simulink model "Sim_CVBT"  (R2022a)
settings: Solver=ode45  StartTime=0.0  StopTime=600  FixedStep=0.01  RelTol=1e-3  EnableMultiTasking=on
InitFcn:
  | initialize;
  | %graphics_init;
values from neighbouring files (symbols this model uses):
  a = 0.08    [initialize.m]
  b = 0.002*0    (= 0)    [initialize.m]
  Kdv = 0    [initialize.m]
  Kiv = 0    [initialize.m]
  Kpsi = 2    [initialize.m]
  Kpv = 0.2    [initialize.m]
  numVeh = 6    [initialize.m]
  P0 = zeros(40,1)    [initialize.m]
  P0tg = [-400 -400 0]    [initialize.m]
  psi0 = zeros(20,1)    [initialize.m]
  rho_d = [100 150 100 150 100 150 100 150 100 150]    [initialize.m]
  Vg = zeros(10,1)    [initialize.m]
  Vmax = 60    [initialize.m]
  Vmin = 10    [initialize.m]
  z0 = zeros(20,1)    [initialize.m]
libraries: slpidlib x6, simulink x2
(part 2 of 2)

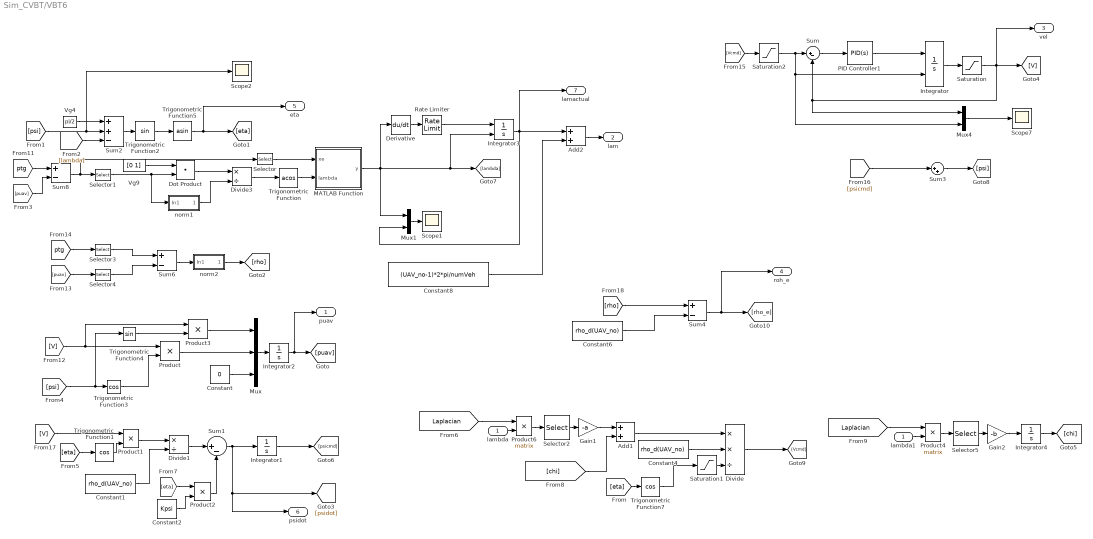
== system Sim_CVBT/VBT6 ==
  lambda : Inport
  Add1 : Sum
  Add2 : Sum
  Constant : Constant  Value=0
  Constant1 : Constant  Value=rho_d(UAV_no)
  Constant2 : Constant  Value=Kpsi
  Constant4 : Constant  Value=rho_d(UAV_no)
  Constant6 : Constant  Value=rho_d(UAV_no)
  Constant8 : Constant  Value=(UAV_no-1)*2*pi/numVeh
  Derivative : Derivative
  Divide : Product  Inputs=**/
  Divide1 : Product  Inputs=*/
  Divide3 : Product  Inputs=*/
  Dot Product : DotProduct  OutDataTypeStr=Inherit: Inherit via internal rule
  Gain1 : Gain  Gain=-a
  Gain2 : Gain  Gain=-b
  Integrator : Integrator  InitialConditionSource=external
  Integrator1 : Integrator  InitialCondition=psi0(UAV_no)*pi/180
  Integrator2 : Integrator  InitialCondition=[P0(2*UAV_no-1) P0(2*UAV_no) z0(UAV_no)]
  Integrator3 : Integrator  InitialConditionSource=external
  Integrator4 : Integrator  InitialCondition=Vg(UAV_no)/rho_d(UAV_no)
  MATLAB Function : MATLAB Function  TreatAsAtomicUnit=on
  Mux : Mux  Inputs=3
  Mux1 : Mux  Inputs=2
  Mux4 : Mux  Inputs=2
  PID Controller1 : slpidlib/PID Controller  Controller=PID  Form=Parallel  TimeDomain=Continuous-time  UseExternalTs=off  SampleTime=1  IntegratorMethod=Forward Euler  FilterMethod=Forward Euler  ControllerParametersSource=internal  P=Kpv  I=Kiv  UseKiTs=off  D=Kdv  N=100  UseFilter=on  TunerSelectOption=Transfer Function Based (PID Tuner App)  InitialConditionSource=internal  InitialConditionForIntegrator=0  InitialConditionForFilter=0  DifferentiatorICPrevScaledInput=0  ExternalReset=none  TrackingMode=off  Kt=1  LimitOutput=off  SatLimitsSource=internal  UpperSaturationLimit=inf  LowerSaturationLimit=-inf  LinearizeAsGain=on  AntiWindupMode=none  Kb=1  POutMin=[]  POutMax=[]  IOutMin=[]  IOutMax=[]  DOutMin=[]  DOutMax=[]  NOutMin=[]  NOutMax=[]  SumOutMin=[]  SumOutMax=[]  SaturationOutMin=[]  SaturationOutMax=[]  PParamMin=[]  PParamMax=[]  IParamMin=[]  IParamMax=[]  DParamMin=[]  DParamMax=[]  NParamMin=[]  NParamMax=[]  KbParamMin=[]  KbParamMax=[]  KtParamMin=[]  KtParamMax=[]  KbOutMin=[]  KbOutMax=[]  KtOutMin=[]  KtOutMax=[]  IntegratorOutMin=[]  IntegratorOutMax=[]  FilterOutMin=[]  FilterOutMax=[]  SumI1OutMin=[]  SumI1OutMax=[]  SumI2OutMin=[]  SumI2OutMax=[]  SumI3OutMin=[]  SumI3OutMax=[]  SumI4OutMin=[]  SumI4OutMax=[]  SumDOutMin=[]  SumDOutMax=[]  DifferentiatorOutMin=[]  DifferentiatorOutMax=[]  FilterDiffOutCoefMin=[]  FilterDiffOutCoefMax=[]  ReciprocalOutMin=[]  ReciprocalOutMax=[]  SumDenOutMin=[]  SumDenOutMax=[]  SumNumOutMin=[]  SumNumOutMax=[]  DivideOutMin=[]  DivideOutMax=[]  UdiffTsProdOutMin=[]  UdiffTsProdOutMax=[]  NTsProdOutMin=[]  NTsProdOutMax=[]  UintegralTsProdOutMin=[]  UintegralTsProdOutMax=[]  UngainTsProdOutMin=[]  UngainTsProdOutMax=[]  IntegratorContinuousStateAttributes=''  IntegratorStateMustResolveToSignalObject=off  IntegratorRTWStateStorageClass=Auto  FilterContinuousStateAttributes=''  FilterStateMustResolveToSignalObject=off  FilterRTWStateStorageClass=Auto  ParallelPVariant=InternalParameters  IdealPVariant=Disabled  IVariant=InternalParameters  DVariant=InternalParameters  IntegratorVariant=Continuous  SatVariant=Disabled  AWVariant=Passthrough  PCopyVariant=Disabled  TRVariant=Disabled  FdbkBlocksVariant=Forward  IdealPFdbkVariant=Disabled  SatFdbkVariant=Disabled  DerivativeFilterVariant=ContFilter  NVariant=InternalParameters  NCopyVariant=Disabled  FilterICVariant=InternalICsFilter  IntegratorICVariant=InternalICs  ExternalResetVariant=Disabled  TRSumVariant=Passthrough  SumFdbkVariant=Disabled  SumVariant=Sum_PID  TsampFilterVariant=InternalTs  TsampNgainVariant=Passthrough  TsampIntegralVariant=Passthrough  ExternalSaturationOutDataTypeStr=Inherit: Same as second input  aMode=0
  Product{,1..3} (4 alike) : Product  RndMeth=Zero
  Product4 : Product  Multiplication=Matrix(*)  RndMeth=Zero
  Product6 : Product  Multiplication=Matrix(*)  RndMeth=Zero
  Rate Limiter : RateLimiter  RisingSlewLimit=100  FallingSlewLimit=-0.1  SampleTimeMode=inherited
  Saturation : Saturate  UpperLimit=Vmax  LowerLimit=Vmin
  Saturation1 : Saturate  UpperLimit=1  LowerLimit=0.8
  Saturation2 : Saturate  UpperLimit=Vmax  LowerLimit=Vmin
  Scope1 : Scope
  Scope2 : Scope
  Scope7 : Scope
  Selector : Selector  InputPortWidth=3  IndexOptions=Index vector (dialog)  Indices=1  OutputSizes=1
  Selector1 : Selector  InputPortWidth=3  IndexOptions=Index vector (dialog)  Indices=[1 2]  OutputSizes=1
  Selector2 : Selector  InputPortWidth=6  IndexOptions=Index vector (dialog)  Indices=[UAV_no]  OutputSizes=1
  Selector3 : Selector  InputPortWidth=3  IndexOptions=Index vector (dialog)  Indices=[1 2]  OutputSizes=1
  Selector4 : Selector  InputPortWidth=3  IndexOptions=Index vector (dialog)  Indices=[1 2]  OutputSizes=1
  Selector5 : Selector  InputPortWidth=6  IndexOptions=Index vector (dialog)  Indices=[UAV_no]  OutputSizes=1
  Sum : Sum  Inputs=|+-
  Sum1 : Sum  Inputs=|+-
  Sum2 : Sum  Inputs=++-
  Sum3 : Sum  Inputs=|++
  Sum4 : Sum  Inputs=+-
  Sum6 : Sum  Inputs=+-
  Sum8 : Sum  Inputs=+-
  Trigonometric Function : Trigonometry  Operator=acos
  Trigonometric Function1 : Trigonometry  Operator=cos
  Trigonometric Function2 : Trigonometry
  Trigonometric Function3 : Trigonometry  Operator=cos
  Trigonometric Function4 : Trigonometry
  Trigonometric Function5 : Trigonometry  Operator=asin
  Trigonometric Function7 : Trigonometry  Operator=cos
  Vg4 : Constant  Value=pi/2
  Vg9 : Constant  Value=[0 1]
  lambda1 : InportShadow
  norm1 : Subsystem
  norm2 : Subsystem
  puav : Outport
  lam : Outport  Port=2
  vel : Outport  Port=3
  roh_e : Outport  Port=4
  eta : Outport  Port=5
  psidot : Outport  Port=6
  lamactual : Outport  Port=7
  wires:
  Mux4/1 -> Scope7/1
  PID Controller1/1 -> Integrator/1
  Integrator/1 -> Saturation/1
  Saturation/1 -> Mux4/1, Sum/2, [V], vel/1
  Saturation1/1 -> Divide/3
  Sum4/1 -> [rho_e], roh_e/1
  Constant6/1 -> Sum4/2
  [rho] -> Sum4/1
  Sum3/1 -> [psi]
  [psicmd] -> Sum3/1
  [Vcmd] -> Saturation2/1
  Sum/1 -> PID Controller1/1
  Constant8/1 -> Add2/2
  Add2/1 -> lam/1
  Integrator3/1 -> lamactual/1, Mux1/2, Add2/1
  Derivative/1 -> Rate Limiter/1
  MATLAB Function/1(y) -> [lambda], Integrator3/2, Mux1/1, Derivative/1
  Divide3/1 -> Trigonometric Function/1
  Trigonometric Function/1 -> MATLAB Function/2(lambda)
  Selector4/1 -> Sum6/2
  Selector3/1 -> Sum6/1
  Selector2/1 -> Gain1/1
  Divide/1 -> [Vcmd]
  lambda/1 -> Product6/2
  [Laplacian] -> Product6/1
  Product6/1 -> Selector2/1
  Constant4/1 -> Divide/2
  Trigonometric Function7/1 -> Saturation1/1
  Gain1/1 -> Add1/1
  Add1/1 -> Divide/1
  [eta] -> Trigonometric Function7/1
  Mux1/1 -> Scope1/1
  [V] -> Product1/1
  norm2/1(Out1) -> [rho]
  Selector1/1 -> norm1/1(In1), Dot Product/2
  Integrator2/1 -> [puav], puav/1
  Mux/1 -> Integrator2/1
  Constant/1 -> Mux/3
  Product/1 -> Mux/2
  Product3/1 -> Mux/1
  Trigonometric Function4/1 -> Product3/2
  Trigonometric Function3/1 -> Product/2
  [psi] -> Trigonometric Function4/1, Trigonometric Function3/1
  [V] -> Product3/1, Product/1
  Trigonometric Function5/1 -> [eta], eta/1
  Trigonometric Function2/1 -> Trigonometric Function5/1
  Vg9/1 -> Dot Product/1
  Selector/1 -> MATLAB Function/1(xe)
  Integrator1/1 -> [psicmd]
  [puav] -> Sum8/2
  [ptg] -> Sum8/1
  norm1/1(Out1) -> Divide3/2
  Dot Product/1 -> Divide3/1
  [lambda] -> Sum2/3
  [psi] -> Sum2/2, Scope2/1
  Sum8/1 -> Selector1/1, Selector/1
  Vg4/1 -> Sum2/1
  Sum2/1 -> Trigonometric Function2/1
  [ptg] -> Selector3/1
  [puav] -> Selector4/1
  Sum6/1 -> norm2/1(In1)
  Sum1/1 -> [psidot], psidot/1, Integrator1/1
  Constant2/1 -> Product2/2
  Product2/1 -> Sum1/2
  [eta] -> Product2/1
  Constant1/1 -> Divide1/2
  Product1/1 -> Divide1/1
  Divide1/1 -> Sum1/1
  [eta] -> Trigonometric Function1/1
  Trigonometric Function1/1 -> Product1/2
  Rate Limiter/1 -> Integrator3/1
  [chi] -> Add1/2
  Selector5/1 -> Gain2/1
  lambda1/1 -> Product4/2
  [Laplacian] -> Product4/1
  Product4/1 -> Selector5/1
  Gain2/1 -> Integrator4/1
  Integrator4/1 -> [chi]
  Saturation2/1 -> Sum/1, Integrator/2, Mux4/2

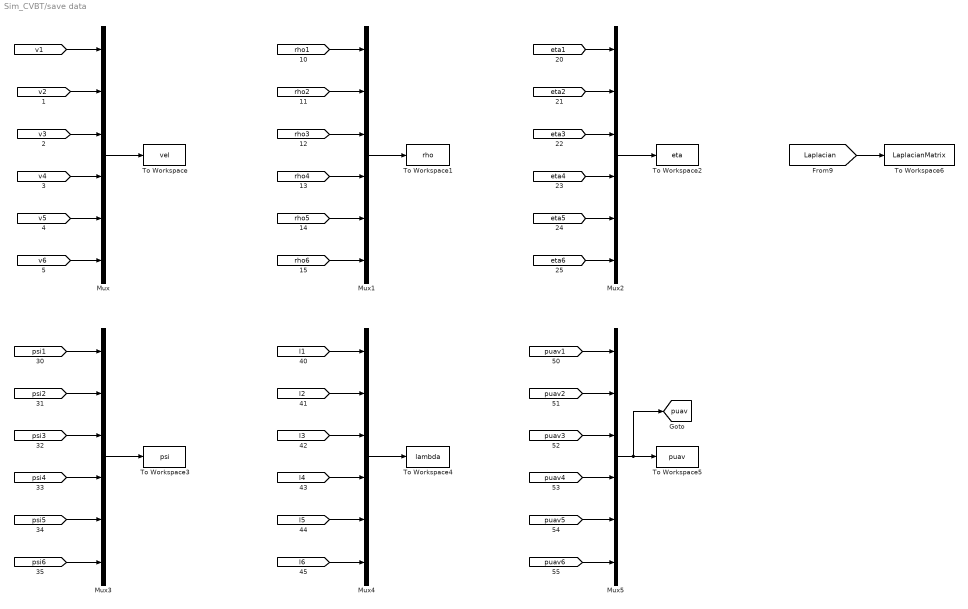
== system Sim_CVBT/save data ==
  Mux{,1..5} (6 alike) : Mux  Inputs=6
  To Workspace : ToWorkspace  VariableName=vel  SaveFormat=Timeseries  SampleTime=-1
  To Workspace1 : ToWorkspace  VariableName=rho  SaveFormat=Timeseries  SampleTime=-1
  To Workspace2 : ToWorkspace  VariableName=eta  SaveFormat=Timeseries  SampleTime=-1
  To Workspace3 : ToWorkspace  VariableName=psi  SaveFormat=Timeseries  SampleTime=-1
  To Workspace4 : ToWorkspace  VariableName=lambda  SaveFormat=Timeseries  SampleTime=-1
  To Workspace5 : ToWorkspace  VariableName=puav  SaveFormat=Timeseries  SampleTime=-1
  To Workspace6 : ToWorkspace  VariableName=LaplacianMatrix  SaveFormat=Timeseries  SampleTime=-1
  tag scope: puav=global
  wires:
  [v1] -> Mux/1
  [v3] -> Mux/3
  [v6] -> Mux/6
  [v5] -> Mux/5
  [v4] -> Mux/4
  [v2] -> Mux/2
  [rho3] -> Mux1/3
  [rho6] -> Mux1/6
  [rho5] -> Mux1/5
  [rho4] -> Mux1/4
  [rho2] -> Mux1/2
  [rho1] -> Mux1/1
  [eta3] -> Mux2/3
  [eta6] -> Mux2/6
  [eta5] -> Mux2/5
  [eta4] -> Mux2/4
  [eta2] -> Mux2/2
  [eta1] -> Mux2/1
  [psi3] -> Mux3/3
  [psi6] -> Mux3/6
  [psi5] -> Mux3/5
  [psi4] -> Mux3/4
  [psi2] -> Mux3/2
  [psi1] -> Mux3/1
  [l3] -> Mux4/3
  [l6] -> Mux4/6
  [l5] -> Mux4/5
  [l4] -> Mux4/4
  [l2] -> Mux4/2
  [l1] -> Mux4/1
  Mux/1 -> To Workspace/1
  Mux1/1 -> To Workspace1/1
  Mux2/1 -> To Workspace2/1
  Mux3/1 -> To Workspace3/1
  Mux4/1 -> To Workspace4/1
  [puav3] -> Mux5/3
  [puav6] -> Mux5/6
  [puav5] -> Mux5/5
  [puav4] -> Mux5/4
  [puav2] -> Mux5/2
  [puav1] -> Mux5/1
  Mux5/1 -> [puav], To Workspace5/1
  [Laplacian] -> To Workspace6/1

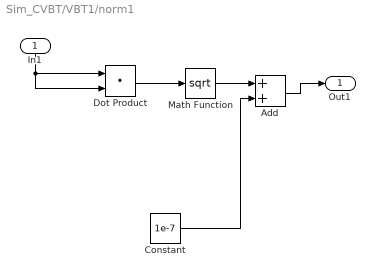
== system Sim_CVBT/VBT1/norm1 ==
  In1 : Inport
  Add : Sum
  Constant : Constant  Value=1e-7
  Dot Product : DotProduct  OutDataTypeStr=Inherit: Inherit via internal rule
  Math Function : Math  Operator=sqrt  SignedPower=on
  Out1 : Outport
  wires:
  Dot Product/1 -> Math Function/1
  In1/1 -> Dot Product/1, Dot Product/2
  Math Function/1 -> Add/1
  Constant/1 -> Add/2
  Add/1 -> Out1/1

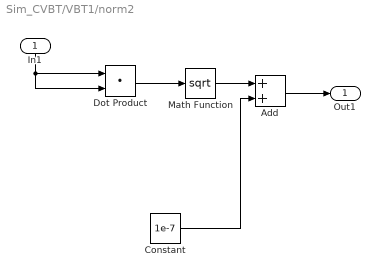
== system Sim_CVBT/VBT1/norm2 ==
  In1 : Inport
  Add : Sum
  Constant : Constant  Value=1e-7
  Dot Product : DotProduct  OutDataTypeStr=Inherit: Inherit via internal rule
  Math Function : Math  Operator=sqrt  SignedPower=on
  Out1 : Outport
  wires:
  Add/1 -> Out1/1
  Constant/1 -> Add/2
  Math Function/1 -> Add/1
  In1/1 -> Dot Product/2, Dot Product/1
  Dot Product/1 -> Math Function/1

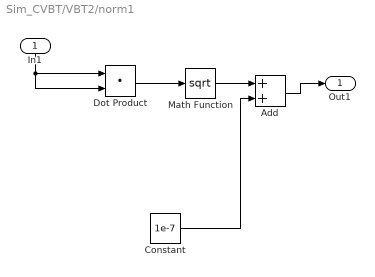
== system Sim_CVBT/VBT2/norm1 ==
  In1 : Inport
  Add : Sum
  Constant : Constant  Value=1e-7
  Dot Product : DotProduct  OutDataTypeStr=Inherit: Inherit via internal rule
  Math Function : Math  Operator=sqrt  SignedPower=on
  Out1 : Outport
  wires:
  Add/1 -> Out1/1
  Constant/1 -> Add/2
  Math Function/1 -> Add/1
  In1/1 -> Dot Product/2, Dot Product/1
  Dot Product/1 -> Math Function/1

== system Sim_CVBT/VBT2/norm2 ==
  In1 : Inport
  Add : Sum
  Constant : Constant  Value=1e-7
  Dot Product : DotProduct  OutDataTypeStr=Inherit: Inherit via internal rule
  Math Function : Math  Operator=sqrt  SignedPower=on
  Out1 : Outport
  wires:
  Dot Product/1 -> Math Function/1
  In1/1 -> Dot Product/1, Dot Product/2
  Math Function/1 -> Add/1
  Constant/1 -> Add/2
  Add/1 -> Out1/1

== system Sim_CVBT/VBT3/norm1 ==
  In1 : Inport
  Add : Sum
  Constant : Constant  Value=1e-7
  Dot Product : DotProduct  OutDataTypeStr=Inherit: Inherit via internal rule
  Math Function : Math  Operator=sqrt  SignedPower=on
  Out1 : Outport
  wires:
  Dot Product/1 -> Math Function/1
  In1/1 -> Dot Product/1, Dot Product/2
  Math Function/1 -> Add/1
  Constant/1 -> Add/2
  Add/1 -> Out1/1

== system Sim_CVBT/VBT3/norm2 ==
  In1 : Inport
  Add : Sum
  Constant : Constant  Value=1e-7
  Dot Product : DotProduct  OutDataTypeStr=Inherit: Inherit via internal rule
  Math Function : Math  Operator=sqrt  SignedPower=on
  Out1 : Outport
  wires:
  Add/1 -> Out1/1
  Constant/1 -> Add/2
  Math Function/1 -> Add/1
  In1/1 -> Dot Product/2, Dot Product/1
  Dot Product/1 -> Math Function/1

== system Sim_CVBT/VBT4/norm1 ==
  In1 : Inport
  Add : Sum
  Constant : Constant  Value=1e-7
  Dot Product : DotProduct  OutDataTypeStr=Inherit: Inherit via internal rule
  Math Function : Math  Operator=sqrt  SignedPower=on
  Out1 : Outport
  wires:
  Add/1 -> Out1/1
  Constant/1 -> Add/2
  Math Function/1 -> Add/1
  In1/1 -> Dot Product/2, Dot Product/1
  Dot Product/1 -> Math Function/1

== system Sim_CVBT/VBT4/norm2 ==
  In1 : Inport
  Add : Sum
  Constant : Constant  Value=1e-7
  Dot Product : DotProduct  OutDataTypeStr=Inherit: Inherit via internal rule
  Math Function : Math  Operator=sqrt  SignedPower=on
  Out1 : Outport
  wires:
  Dot Product/1 -> Math Function/1
  In1/1 -> Dot Product/1, Dot Product/2
  Math Function/1 -> Add/1
  Constant/1 -> Add/2
  Add/1 -> Out1/1

== system Sim_CVBT/VBT5/norm1 ==
  In1 : Inport
  Add : Sum
  Constant : Constant  Value=1e-7
  Dot Product : DotProduct  OutDataTypeStr=Inherit: Inherit via internal rule
  Math Function : Math  Operator=sqrt  SignedPower=on
  Out1 : Outport
  wires:
  Dot Product/1 -> Math Function/1
  In1/1 -> Dot Product/1, Dot Product/2
  Math Function/1 -> Add/1
  Constant/1 -> Add/2
  Add/1 -> Out1/1

== system Sim_CVBT/VBT5/norm2 ==
  In1 : Inport
  Add : Sum
  Constant : Constant  Value=1e-7
  Dot Product : DotProduct  OutDataTypeStr=Inherit: Inherit via internal rule
  Math Function : Math  Operator=sqrt  SignedPower=on
  Out1 : Outport
  wires:
  Add/1 -> Out1/1
  Constant/1 -> Add/2
  Math Function/1 -> Add/1
  In1/1 -> Dot Product/2, Dot Product/1
  Dot Product/1 -> Math Function/1

== system Sim_CVBT/VBT6/norm1 ==
  In1 : Inport
  Add : Sum
  Constant : Constant  Value=1e-7
  Dot Product : DotProduct  OutDataTypeStr=Inherit: Inherit via internal rule
  Math Function : Math  Operator=sqrt  SignedPower=on
  Out1 : Outport
  wires:
  Add/1 -> Out1/1
  Constant/1 -> Add/2
  Math Function/1 -> Add/1
  In1/1 -> Dot Product/2, Dot Product/1
  Dot Product/1 -> Math Function/1

== system Sim_CVBT/VBT6/norm2 ==
  In1 : Inport
  Add : Sum
  Constant : Constant  Value=1e-7
  Dot Product : DotProduct  OutDataTypeStr=Inherit: Inherit via internal rule
  Math Function : Math  Operator=sqrt  SignedPower=on
  Out1 : Outport
  wires:
  Dot Product/1 -> Math Function/1
  In1/1 -> Dot Product/1, Dot Product/2
  Math Function/1 -> Add/1
  Constant/1 -> Add/2
  Add/1 -> Out1/1

== matlab function Sim_CVBT/VBT1/MATLAB Function ==
  data: xe input; y output; lambda input
function y = fcn(xe,lambda)
u=lambda;
if xe > 0 
    u = lambda;
else
    u = 2*pi-lambda;
end
y = u;

== matlab function Sim_CVBT/VBT2/MATLAB Function ==
  data: xe input; y output; lambda input
function y = fcn(xe,lambda)
u=lambda;
if xe > 0 
    u = lambda;
else
    u = 2*pi-lambda;
end
y = u;

== matlab function Sim_CVBT/VBT3/MATLAB Function ==
  data: xe input; y output; lambda input
function y = fcn(xe,lambda)
u=lambda;
if xe > 0 
    u = lambda;
else
    u = 2*pi-lambda;
end
y = u;

== matlab function Sim_CVBT/VBT4/MATLAB Function ==
  data: xe input; y output; lambda input
function y = fcn(xe,lambda)
u=lambda;
if xe > 0 
    u = lambda;
else
    u = 2*pi-lambda;
end
y = u;

== matlab function Sim_CVBT/VBT5/MATLAB Function ==
  data: xe input; y output; lambda input
function y = fcn(xe,lambda)
u=lambda;
if xe > 0 
    u = lambda;
else
    u = 2*pi-lambda;
end
y = u;

== matlab function Sim_CVBT/VBT6/MATLAB Function ==
  data: xe input; y output; lambda input
function y = fcn(xe,lambda)
u=lambda;
if xe > 0 
    u = lambda;
else
    u = 2*pi-lambda;
end
y = u;

== matlab function Sim_CVBT/MATLAB Function1 ==
  data: xy input; Laplacian output; numVeh parameter
function Laplacian = fcn(xy,numVeh)
a = zeros(6);
Laplacian = zeros(6);
for i = 1:numVeh
    for j = i+1:numVeh
        if sqrt((xy(2*i-1)-xy(2*j-1))^2+(xy(2*i)-xy(2*j))^2) < 250
            a(i,j) = -1;
            a(j,i) = -1;
            a(i,i) = a(i,i)+1;
            a(j,j) = a(j,j)+1;
        end
    end
end


Laplacian = a;
